simulink model "Hw1_ME8352sim"  (R2020b)
settings: Solver=VariableStepAuto  StartTime=0.0  StopTime=t_sim  RelTol=1e-5
values from neighbouring files (symbols this model uses):
  c = 3    [Hw1_ME8352.m]
  k = 2    [Hw1_ME8352.m]
  m = 1    [Hw1_ME8352.m]
  step_val = step_array(i)    [Hw1_ME8352.m]
  vdot0 = 1.5    [Hw1_ME8352.m]
  x_0 = x0_array(i)    [Hw1_ME8352.m]
  x_dot0 = xdot0_array(ii)    [Hw1_ME8352.m]
settings Model: Creator=dempseca  LastModifiedBy=dempseca

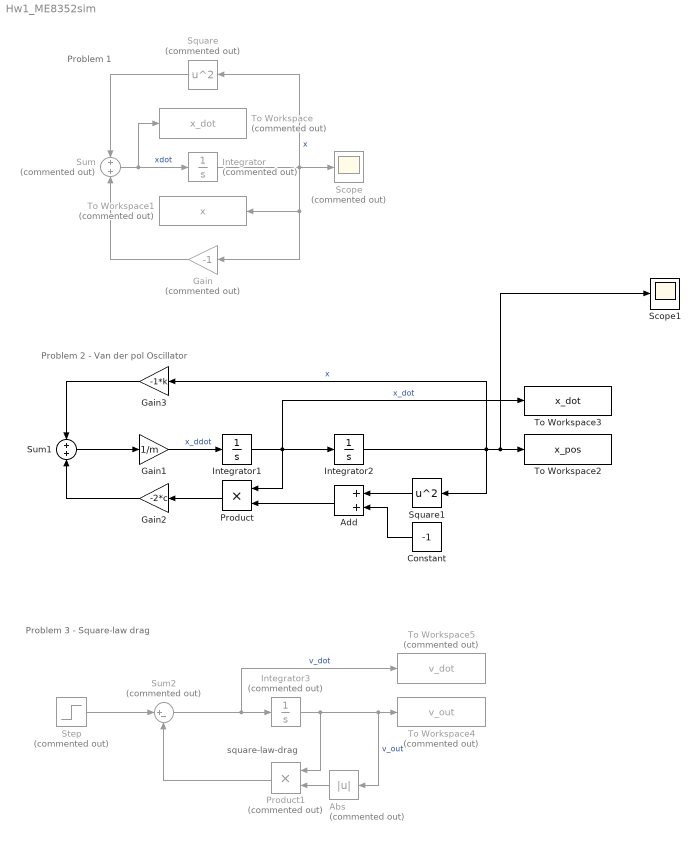
== system Hw1_ME8352sim ==
  note: Problem 3 - Square-law drag
  note: square-law-drag
  note: Problem 2 - Van der pol Oscillator
  note: Problem 1
  Abs : Abs  Commented=on
  Add : Sum
  Constant : Constant  Value=-1
  Gain : Gain  Commented=on  Gain=-1
  Gain1 : Gain  Gain=1/m
  Gain2 : Gain  Gain=-2*c
  Gain3 : Gain  Gain=-1*k
  Integrator : Integrator  Commented=on  InitialCondition=x_dot0
  Integrator1 : Integrator  InitialCondition=x_dot0
  Integrator2 : Integrator  InitialCondition=x_0
  Integrator3 : Integrator  Commented=on  InitialCondition=vdot0
  Product : Product
  Product1 : Product  Commented=on
  Scope : Scope  Commented=on
  Scope1 : Scope
  Square : Math  Commented=on  Operator=square  SaturateOnIntegerOverflow=on
  Square1 : Math  Operator=square  SaturateOnIntegerOverflow=on
  Step : Step  Commented=on  Time=0  After=step_val  SampleTime=0
  Sum : Sum  Commented=on
  Sum1 : Sum
  Sum2 : Sum  Commented=on  Inputs=|+-
  To Workspace : ToWorkspace  Commented=on  VariableName=x_dot  SaveFormat=Timeseries  SampleTime=-1
  To Workspace1 : ToWorkspace  Commented=on  VariableName=x  SaveFormat=Timeseries  SampleTime=-1
  To Workspace2 : ToWorkspace  VariableName=x_pos  SaveFormat=Timeseries  SampleTime=-1
  To Workspace3 : ToWorkspace  VariableName=x_dot  SaveFormat=Timeseries  SampleTime=-1
  To Workspace4 : ToWorkspace  Commented=on  VariableName=v_out  SaveFormat=Timeseries  SampleTime=-1
  To Workspace5 : ToWorkspace  Commented=on  VariableName=v_dot  SaveFormat=Timeseries  SampleTime=-1
  wires:
  Integrator/1 -> To Workspace1/1, Gain/1, Square/1, Scope/1  "x"
  Sum/1 -> To Workspace/1, Integrator/1  "xdot"
  Gain/1 -> Sum/2
  Square/1 -> Sum/1
  Integrator1/1 -> To Workspace3/1, Product/1, Integrator2/1  "x_dot"
  Gain1/1 -> Integrator1/1  "x_ddot"
  Integrator2/1 -> Gain3/1, Square1/1, Scope1/1, To Workspace2/1  "x"
  Sum1/1 -> Gain1/1
  Square1/1 -> Add/1
  Constant/1 -> Add/2
  Add/1 -> Product/2
  Product/1 -> Gain2/1
  Gain2/1 -> Sum1/2
  Gain3/1 -> Sum1/1
  Integrator3/1 -> Product1/1, Abs/1, To Workspace4/1  "v_out"
  Sum2/1 -> To Workspace5/1, Integrator3/1  "v_dot"
  Step/1 -> Sum2/1
  Abs/1 -> Product1/2
  Product1/1 -> Sum2/2
